simulink model "condom"  (R2015a)
settings: Solver=ode45  StartTime=0.0  StopTime=10.0  RelTol=1e-3
libraries: simulink x4
settings Model: Creator=GSavaia  LastModifiedBy=GSavaia

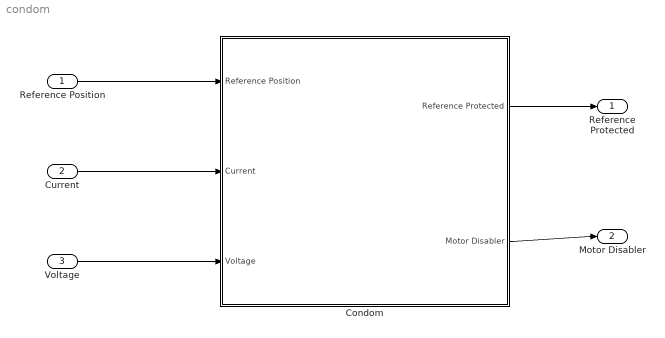
== system condom ==
  Reference Position : Inport
  "Current " : Inport  Port=2
  Voltage : Inport  Port=3
  Condom : Subsystem
  Reference Protected : Outport
  Motor Disabler : Outport  Port=2
  wires:
  Reference Position/1 -> Condom/1(Reference Position)
  "Current "/1 -> Condom/2("Current ")
  Voltage/1 -> Condom/3(Voltage)
  Condom/1(Reference Protected) -> Reference Protected/1
  Condom/2(Motor Disabler) -> Motor Disabler/1

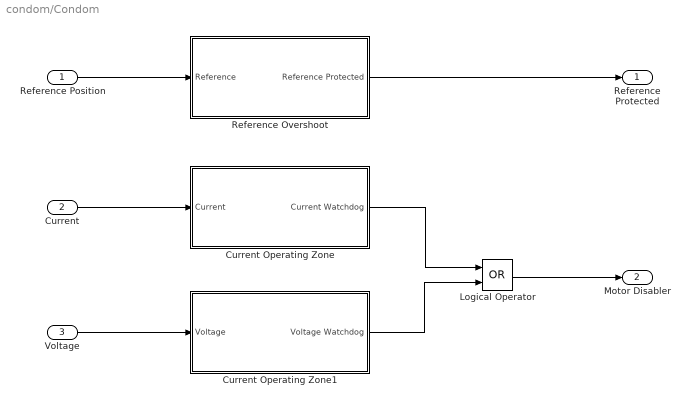
== system condom/Condom ==
  Reference Position : Inport
  "Current " : Inport  Port=2
  Voltage : Inport  Port=3
  Current Operating Zone : Subsystem
  Current Operating Zone1 : Subsystem
  Logical Operator : Logic  Operator=OR  AllPortsSameDT=off  OutDataTypeStr=boolean
  Reference Overshoot : Subsystem
  Reference Protected : Outport
  Motor Disabler : Outport  Port=2
  wires:
  Reference Overshoot/1(Reference Protected) -> Reference Protected/1
  "Current "/1 -> Current Operating Zone/1(Current)
  Reference Position/1 -> Reference Overshoot/1("Reference ")
  Voltage/1 -> Current Operating Zone1/1(Voltage)
  Logical Operator/1 -> Motor Disabler/1
  Current Operating Zone/1(Current Watchdog) -> Logical Operator/1
  Current Operating Zone1/1(Voltage Watchdog) -> Logical Operator/2

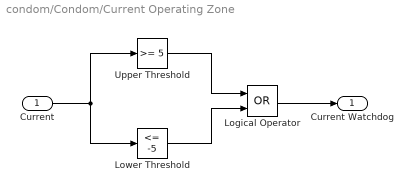
== system condom/Condom/Current Operating Zone ==
  Current : Inport
  Logical Operator : Logic  Operator=OR  AllPortsSameDT=off  OutDataTypeStr=boolean
  Lower Threshold : simulink/Logic and Bit Operations/Compare To Constant  relop=<=  const=-5  OutDataTypeStr=boolean
  Upper Threshold : simulink/Logic and Bit Operations/Compare To Constant  relop=>=  const=5  OutDataTypeStr=boolean
  Current Watchdog : Outport
  wires:
  Current/1 -> Lower Threshold/1, Upper Threshold/1
  Logical Operator/1 -> Current Watchdog/1
  Upper Threshold/1 -> Logical Operator/1
  Lower Threshold/1 -> Logical Operator/2

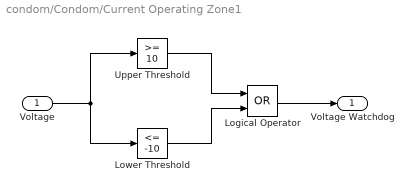
== system condom/Condom/Current Operating Zone1 ==
  Voltage : Inport
  Logical Operator : Logic  Operator=OR  AllPortsSameDT=off  OutDataTypeStr=boolean
  Lower Threshold : simulink/Logic and Bit Operations/Compare To Constant  relop=<=  const=-10  OutDataTypeStr=boolean
  Upper Threshold : simulink/Logic and Bit Operations/Compare To Constant  relop=>=  const=10  OutDataTypeStr=boolean
  Voltage Watchdog : Outport
  wires:
  Voltage/1 -> Lower Threshold/1, Upper Threshold/1
  Logical Operator/1 -> Voltage Watchdog/1
  Upper Threshold/1 -> Logical Operator/1
  Lower Threshold/1 -> Logical Operator/2

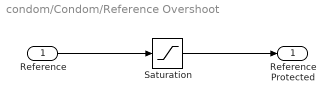
== system condom/Condom/Reference Overshoot ==
  "Reference " : Inport
  Saturation : Saturate  UpperLimit=3  LowerLimit=-3
  Reference Protected : Outport
  wires:
  "Reference "/1 -> Saturation/1
  Saturation/1 -> Reference Protected/1
